simulink model "TesteNucleo"  (R2018b)
settings: Solver=FixedStepAuto  StartTime=0.0  StopTime=200.0  RelTol=1e-3  EnableMultiTasking=on
libraries: mbedblockslib x6
settings Model: ExtModeTrigDuration=10  Creator=victo  LastModifiedBy=victo
settings OptimizationCC: EnhancedBackFolding=on  PassReuseOutputArgsAs=Individual arguments  MaxStackSize=64  OptimizeBlockOrder=speed  DifferentSizesBufferReuse=on  OptimizationCustomize=off
settings DebuggingCC: ParameterTunabilityLossMsg=error
settings HardwareCC: ProdBitPerPointer=32  ProdBitPerSizeT=32  ProdBitPerPtrDiffT=32  ProdLargestAtomicInteger=Long  ProdLargestAtomicFloat=Double  ProdWordSize=32  ProdHWDeviceType=ARM Compatible->ARM Cortex
settings SFSimCC: MATLABDynamicMemAlloc=off
settings RTWCC: SystemTargetFile=ert.tlc  HardwareBoard=STM32 Nucleo F767ZI  TemplateMakefile=ert_default_tmf  GenerateReport=on  Toolchain=GNU Tools for ARM Embedded Processors  IncludeHyperlinkInReport=on  LaunchReport=on  GenerateTraceInfo=on  GenerateTraceReport=on  GenerateTraceReportSl=on  GenerateTraceReportSf=on  GenerateTraceReportEml=on
settings CodeAppCC: ForceParamTrailComments=on  IgnoreCustomStorageClasses=off  OperatorAnnotations=on  SimulinkDataObjDesc=on  SFDataObjDesc=on  InsertBlockDesc=on

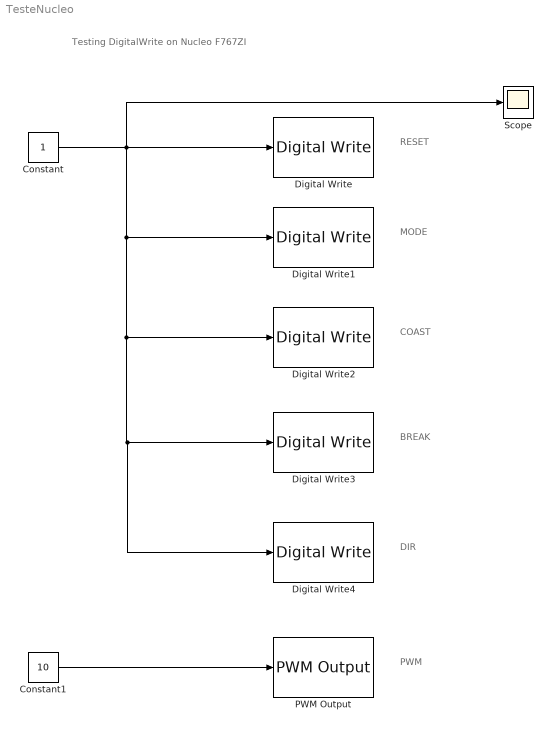
== system TesteNucleo ==
  note: Testing DigitalWrite on Nucleo F767ZI
  note: RESET
  note: MODE
  note: COAST
  note: BREAK
  note: DIR
  note: PWM
  Constant : Constant
  Constant1 : Constant  Value=10
  Digital Write : mbedblockslib/Digital Write  Pin=PE_15  Direction=output
      settings: SourceProductName=Simulink Coder Support Package for BBC microbit Board  SourceProductBaseCode=MICROBIT
  Digital Write1 : mbedblockslib/Digital Write  Pin=PE_14  Direction=output
      settings: SourceProductName=Simulink Coder Support Package for BBC microbit Board  SourceProductBaseCode=MICROBIT
  Digital Write2 : mbedblockslib/Digital Write  Pin=PE_12  Direction=output
      settings: SourceProductName=Simulink Coder Support Package for BBC microbit Board  SourceProductBaseCode=MICROBIT
  Digital Write3 : mbedblockslib/Digital Write  Pin=PE_10  Direction=output
      settings: SourceProductName=Simulink Coder Support Package for BBC microbit Board  SourceProductBaseCode=MICROBIT
  Digital Write4 : mbedblockslib/Digital Write  Pin=PB_8  Direction=output
      settings: SourceProductName=Simulink Coder Support Package for BBC microbit Board  SourceProductBaseCode=MICROBIT
  PWM Output : mbedblockslib/PWM Output  Pin=PB_9  EnableInputFrequency=off  InitialFrequency=20000  InitialDutyCycle=10  NotificationType=None
      settings: SourceProductName=Simulink Coder Support Package for BBC microbit Board  SourceProductBaseCode=MICROBIT
  Scope : Scope
  wires:
  Constant/1 -> Digital Write4/1, Digital Write3/1, Digital Write2/1, Digital Write1/1, Scope/1, Digital Write/1
  Constant1/1 -> PWM Output/1
